simulink model "Lateral_Contrl_with_MPC"  (R2021a)
settings: Solver=VariableStepAuto  StartTime=0.0  StopTime=Ts  RelTol=1e-3
InitFcn:
  | Lateral_Control_with_MPC
StopFcn:
  | Lateral_Control_with_MPC_simulation_plot
values from neighbouring files (symbols this model uses):
  Vx = 30    [Lateral_Control_with_MPC.m]
libraries: mpclib x1
settings Model: Creator=User  LastModifiedBy=User

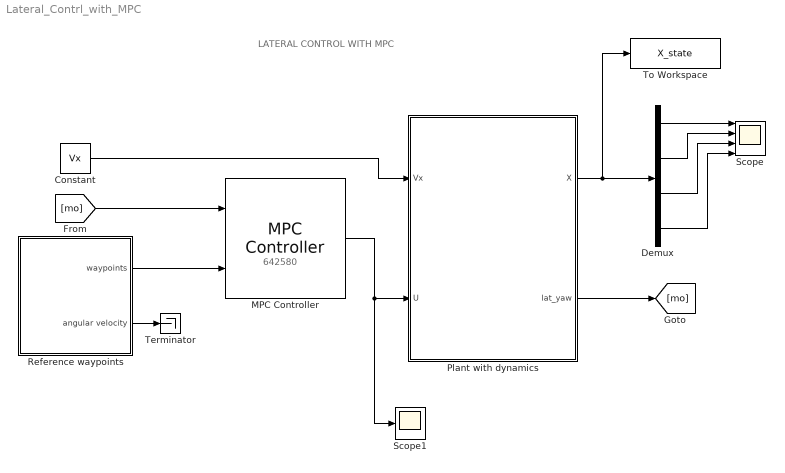
== system Lateral_Contrl_with_MPC ==
  note: 642580
  note: LATERAL CONTROL WITH MPC
  Constant : Constant  Value=Vx
  Demux : Demux
  MPC Controller : mpclib/MPC Controller  SCDEnableBlockLinearizationSpecification=on  mpcobj=mpc1  is_multiple=0  enable_value=0  return_u0=off  updateMPCinCallerWorkspace=on  md_inport=off  mv_inport=off  uref_inport=off  return_cost=off  return_mvseq=off  return_qpstatus=off  return_xseq=off  return_state=off  return_ovseq=off  state_inport=off  umin_inport=off  umax_inport=off  ymin_inport=off  ymax_inport=off  cc_inport=off  ywt_inport=off  uwt_inport=off  duwt_inport=off  rhoeps_inport=off  pm_inport=off  MaximumP=10  HorizonChoice=FixedHorizon  n_ts=0.1  n_p=10  n_mv=1  n_md=0  n_ud=0  n_mo=2  n_uo=0  BlockDataType=double  SampleTimeInherited=off  switch_inport=off
  Plant with dynamics : Subsystem
  Reference waypoints : Subsystem
  Scope : Scope  NumInputPorts=4
  Scope1 : Scope
  Terminator : Terminator
  To Workspace : ToWorkspace  VariableName=X_state  SampleTime=-1
  wires:
  [mo] -> MPC Controller/1
  Constant/1 -> Plant with dynamics/1(Vx)
  Reference waypoints/2(angular velocity) -> Terminator/1
  MPC Controller/1 -> Plant with dynamics/2(U), Scope1/1
  Plant with dynamics/1(X) -> To Workspace/1, Demux/1
  Demux/4 -> Scope/4
  Demux/2 -> Scope/2
  Demux/3 -> Scope/3
  Reference waypoints/1(waypoints) -> MPC Controller/2
  Plant with dynamics/2(lat_yaw) -> [mo]
  Demux/1 -> Scope/1

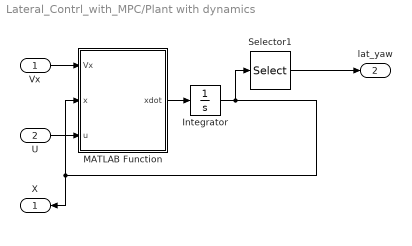
== system Lateral_Contrl_with_MPC/Plant with dynamics ==
  Vx : Inport
  U : Inport  Port=2
  Integrator : Integrator
  MATLAB Function : MATLAB Function  TreatAsAtomicUnit=on
  Selector1 : Selector  InputPortWidth=4  IndexOptions=Index vector (dialog)  Indices=[4 2]  OutputSizes=1
  X : Outport  VectorParamsAs1DForOutWhenUnconnected=off
  lat_yaw : Outport  Port=2  VectorParamsAs1DForOutWhenUnconnected=off
  wires:
  Selector1/1 -> lat_yaw/1
  MATLAB Function/1(xdot) -> Integrator/1
  Integrator/1 -> Selector1/1, MATLAB Function/2(x), X/1
  U/1 -> MATLAB Function/3(u)
  Vx/1 -> MATLAB Function/1(Vx)

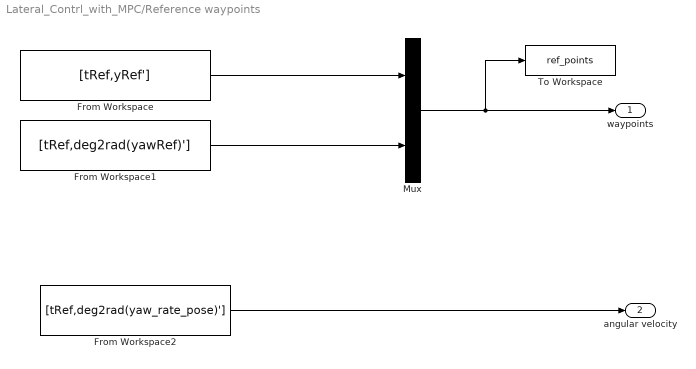
== system Lateral_Contrl_with_MPC/Reference waypoints ==
  From Workspace : FromWorkspace  VariableName=[tRef,yRef']  SampleTime=0.1
  From Workspace1 : FromWorkspace  VariableName=[tRef,deg2rad(yawRef)']  SampleTime=0.1
  From Workspace2 : FromWorkspace  VariableName=[tRef,deg2rad(yaw_rate_pose)']  SampleTime=0.1
  Mux : Mux  Inputs=2
  To Workspace : ToWorkspace  VariableName=ref_points  SampleTime=-1
  waypoints : Outport
  angular velocity : Outport  Port=2
  wires:
  Mux/1 -> To Workspace/1, waypoints/1
  From Workspace/1 -> Mux/1
  From Workspace1/1 -> Mux/2
  From Workspace2/1 -> angular velocity/1

== matlab function Lateral_Contrl_with_MPC/Plant with dynamics/MATLAB Function ==
  data: Vx input; x input size=[4,1]; u input; xdot output size=[4,1]
function xdot = fcn(Vx,x,u)

% Model parameters
m = 1575;
Iz = 2875;
lf = 1.2;
lr = 1.6;
Cf = 19000;
Cr = 33000;

% Continuous-time model
A = [-(2*Cf+2*Cr)/m/Vx, 0, -Vx-(2*Cf*lf-2*Cr*lr)/m/Vx, 0;
     0, 0, 1, 0;
     -(2*Cf*lf-2*Cr*lr)/Iz/Vx, 0, -(2*Cf*lf^2+2*Cr*lr^2)/Iz/Vx, 0;
     1, Vx, 0, 0];
B = [2*Cf/m 0 2*Cf*lf/Iz 0]';   
C = [0 0 0 1; 0 1 0 0];
D = zeros(2,1);
xdot = A*x + B*u;
%y = C*x + D*u;
